simulink model "sampleModel1507_5_sub"  (R2023a)
settings: Solver=VariableStepAuto  StartTime=0.0  StopTime=10.0  RelTol=1e-3
libraries: hdlsllib x8, simulink x3
settings Model: Creator=user1  LastModifiedBy=user1
settings OptimizationCC: BlockReduction=off  ConditionallyExecuteInputs=off

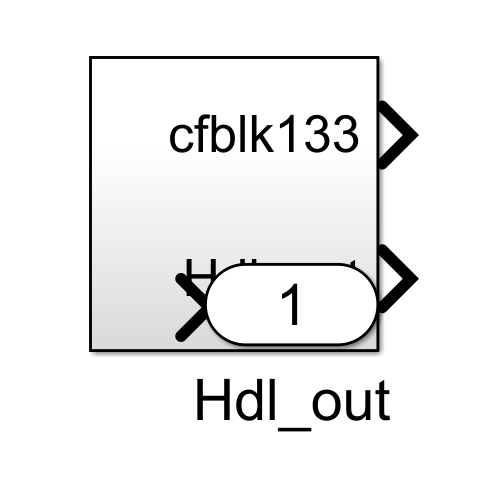
[thumbnail: Simulink's stored preview of the top-level diagram]
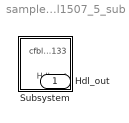
== system sampleModel1507_5_sub ==
  Subsystem : Subsystem
  Hdl_out : Outport  OutDataTypeStr=uint8

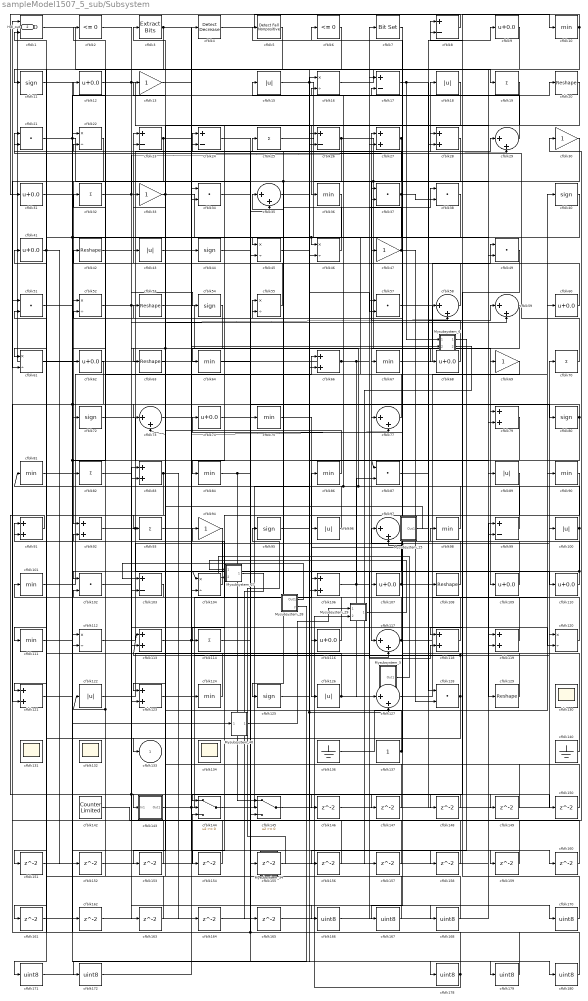
== system sampleModel1507_5_sub/Subsystem ==
  Mysubsystem_15 : Subsystem  TreatAsAtomicUnit=on  RTWFcnName=Mysubsystem_15
      settings: RTWFcnNameOpts=User specified  RTWFileNameOpts=Use function name
  Mysubsystem_27 : Subsystem  TreatAsAtomicUnit=on  RTWFcnName=Mysubsystem_27
      settings: RTWFcnNameOpts=User specified  RTWFileNameOpts=Use function name
  Mysubsystem_28 : Subsystem  TreatAsAtomicUnit=on  RTWFcnName=Mysubsystem_28
      settings: RTWFcnNameOpts=User specified  RTWFileNameOpts=Use function name
  Mysubsystem_29 : Subsystem  TreatAsAtomicUnit=on  RTWFcnName=Mysubsystem_29
      settings: RTWFcnNameOpts=User specified  RTWFileNameOpts=Use function name
  Mysubsystem_34 : Subsystem  TreatAsAtomicUnit=on  RTWFcnName=Mysubsystem_34
      settings: RTWFcnNameOpts=User specified  RTWFileNameOpts=Use function name
  Mysubsystem_40 : Subsystem  TreatAsAtomicUnit=on  RTWFcnName=Mysubsystem_40
      settings: RTWFcnNameOpts=User specified  RTWFileNameOpts=Use function name
  Mysubsystem_5 : Subsystem  TreatAsAtomicUnit=on  RTWFcnName=Mysubsystem_5
      settings: RTWFcnNameOpts=User specified  RTWFileNameOpts=Use function name
  Mysubsystem_6 : Subsystem  TreatAsAtomicUnit=on  RTWFcnName=Mysubsystem_6
      settings: RTWFcnNameOpts=User specified  RTWFileNameOpts=Use function name
  cfblk1 : Logic  AllPortsSameDT=off  OutDataTypeStr=boolean
  cfblk{10,36,64,67,75,81,84,86,90,98,101,111,124} (13 alike) : MinMax  OutDataTypeStr=uint8
  cfblk{15,18,43,89,96,100,122,126} (8 alike) : Abs  OutDataTypeStr=uint8  SaturateOnIntegerOverflow=off
  cfblk{21,34,37..38,49,51,57,87,102,128} (10 alike) : DotProduct  OutDataTypeStr=uint8
  cfblk{8,17,23..24,26,99,103} (7 alike) : Sum  Inputs=+-  OutDataTypeStr=uint8
  cfblk{16,22,45..46,52,55,61,104,112,120} (10 alike) : Product  Inputs=*/  OutDataTypeStr=uint8  RndMeth=Zero  SaturateOnIntegerOverflow=on
  cfblk{27..28,66,79,83,91..92,106,113,118..119,121,123} (13 alike) : Sum  OutDataTypeStr=uint8
  cfblk{9,12,31,41,60,62,68,74,107,109..110,116} (12 alike) : Bias  Bias=0.0  SaturateOnIntegerOverflow=off
  cfblk{20,42,53,63,108,129} (6 alike) : Reshape
  cfblk{11,40,44,54,72,80,95,125} (8 alike) : Signum
  cfblk{19,25,32,70,82,93,114} (7 alike) : Sum  Inputs=+  OutDataTypeStr=uint8
  cfblk{29,35,58..59,73,77,97,117,127} (9 alike) : Sum  Inputs=|++  OutDataTypeStr=uint8
  cfblk{13,30,33,47,69,94} (6 alike) : Gain  OutDataTypeStr=uint8
  cfblk{130..132,134} (4 alike) : Scope
      settings: Floating=on
  cfblk136 : Ground
  cfblk137 : Constant  OutDataTypeStr=uint8  SampleTime=-1
  cfblk140 : Ground
  cfblk142 : hdlsllib/Sources/Counter Limited  uplimit=7  tsamp=-1
  cfblk143 : Subsystem
      settings: LibrarySourceBlock=|
      | hdlsllib/Ports &
      | Subsystems/Subsystem
  cfblk144 : Switch  OutDataTypeStr=uint8  SaturateOnIntegerOverflow=off  InputSameDT=off
  cfblk145 : Switch  OutDataTypeStr=uint8  SaturateOnIntegerOverflow=off  InputSameDT=off
  cfblk{146..165} (20 alike) : Delay  SampleTime=1
  cfblk{166..168,170..172,178..180} (9 alike) : DataTypeConversion  OutDataTypeStr=uint8  SaturateOnIntegerOverflow=off  RndMeth=Floor
  cfblk2 : hdlsllib/Logic and Bit Operations/Compare To Zero  relop=<=  OutDataTypeStr=uint8
  cfblk3 : simulink/Logic and Bit Operations/Extract Bits  bitsToExtract=Upper half  numBits=8  bitIdxRange=[0 7]  outScalingMode=Preserve fixed-point scaling
      settings: LibrarySourceBlock=|
      | hdlsllib/Logic and Bit
      | Operations/Extract Bits
  cfblk4 : simulink/Logic and Bit Operations/Detect Decrease  vinit=0.0  OutDataTypeStr=uint8
      settings: LibrarySourceBlock=|
      | hdlsllib/Logic and Bit
      | Operations/Detect
      | Decrease
  cfblk5 : hdlsllib/Logic and Bit Operations/Detect Fall Nonpositive  vinit=0  OutDataTypeStr=uint8
  cfblk6 : hdlsllib/Logic and Bit Operations/Compare To Zero  relop=<=  OutDataTypeStr=uint8
  cfblk7 : simulink/Logic and Bit Operations/Bit Set  iBit=0
      settings: LibrarySourceBlock=|
      | hdlsllib/Logic and Bit
      | Operations/Bit Set
  cfblk133 : Outport  OutDataTypeStr=uint8  VectorParamsAs1DForOutWhenUnconnected=off
  Hdl_out : Outport  Port=2  OutDataTypeStr=uint8
  wires:
  cfblk67/1 -> cfblk49/1
  cfblk101/1 -> cfblk66/1
  cfblk66/1 -> Hdl_out/1, cfblk38/1, cfblk127/1
  cfblk113/1 -> cfblk158/1, Mysubsystem_6/2(In2)
  cfblk55/1 -> cfblk23/1
  cfblk29/1 -> cfblk15/1
  cfblk99/1 -> cfblk55/2, cfblk64/1
  cfblk83/1 -> cfblk171/1, cfblk164/1
  cfblk26/1 -> cfblk103/2, cfblk79/2, cfblk68/1
  cfblk98/1 -> cfblk16/2, cfblk81/1
  cfblk102/1 -> cfblk166/1, cfblk145/3
  cfblk69/1 -> cfblk45/1
  cfblk47/1 -> cfblk128/2, cfblk21/1
  cfblk38/1 -> cfblk121/1, cfblk46/1
  cfblk57/1 -> cfblk109/1
  cfblk52/1 -> cfblk58/2, cfblk24/1
  cfblk110/1 -> cfblk37/2, cfblk104/1
  cfblk16/1 -> cfblk19/1
  cfblk22/1 -> cfblk92/1
  cfblk92/1 -> cfblk117/2, cfblk18/1
  cfblk100/1 -> cfblk154/1, cfblk37/1
  cfblk145/1 -> cfblk70/1
  cfblk112/1 -> cfblk100/1
  cfblk128/1 -> cfblk161/1, cfblk5/1, cfblk113/1
  cfblk3/1 -> cfblk82/1, cfblk44/1
  cfblk61/1 -> cfblk87/1, Mysubsystem_40/1(In1)
  cfblk80/1 -> cfblk106/2, cfblk72/1
  cfblk129/1 -> cfblk97/2, cfblk42/1
  cfblk75/1 -> cfblk126/1
  cfblk96/1 -> cfblk12/1
  cfblk8/1 -> cfblk31/1
  cfblk70/1 -> cfblk21/2
  cfblk40/1 -> cfblk46/2
  cfblk9/1 -> cfblk66/2
  cfblk116/1 -> cfblk35/1
  cfblk104/1 -> cfblk91/1
  cfblk33/1 -> cfblk73/1, cfblk45/2
  cfblk124/1 -> cfblk32/1
  cfblk127/1 -> cfblk60/1
  cfblk109/1 -> cfblk6/1
  cfblk5/1 -> cfblk11/1
  cfblk123/1 -> cfblk120/1
  cfblk21/1 -> cfblk20/1, cfblk75/1
  cfblk12/1 -> cfblk54/1, cfblk89/1
  cfblk107/1 -> cfblk96/1, cfblk58/1
  cfblk25/1 -> cfblk129/1
  cfblk143/1(Out1) -> cfblk77/2, cfblk86/1
  cfblk20/1 -> cfblk36/1
  cfblk62/1 -> cfblk121/2, cfblk112/2
  cfblk28/1 -> cfblk83/2
  cfblk95/1 -> cfblk168/1
  cfblk97/1 -> cfblk9/1, cfblk102/1
  cfblk126/1 -> cfblk118/2, cfblk41/1
  cfblk15/1 -> cfblk57/2, cfblk117/1
  cfblk18/1 -> cfblk84/1
  cfblk87/1 -> cfblk59/1
  cfblk1/1 -> cfblk99/2
  cfblk89/1 -> cfblk114/1
  cfblk41/1 -> cfblk152/1, cfblk151/1
  cfblk10/1 -> cfblk111/1, cfblk8/1
  cfblk31/1 -> cfblk149/1, cfblk49/2
  cfblk35/1 -> cfblk110/1
  cfblk68/1 -> cfblk27/1
  cfblk91/1 -> cfblk143/1(In1)
  cfblk43/1 -> cfblk4/1
  cfblk27/1 -> cfblk77/1, cfblk125/1, cfblk133/1
  cfblk74/1 -> cfblk116/1
  cfblk63/1 -> cfblk13/1
  cfblk118/1 -> cfblk94/1
  cfblk6/1 -> cfblk61/1
  cfblk17/1 -> cfblk108/1, Mysubsystem_6/1(In1)
  cfblk82/1 -> cfblk113/2
  cfblk19/1 -> cfblk63/1
  cfblk122/1 -> cfblk57/1
  cfblk144/1 -> cfblk26/2
  cfblk108/1 -> cfblk74/1
  cfblk86/1 -> cfblk52/2
  cfblk120/1 -> cfblk106/1
  cfblk58/1 -> cfblk25/1
  cfblk103/1 -> cfblk102/2
  cfblk72/1 -> cfblk119/2
  cfblk119/1 -> cfblk55/1
  cfblk51/1 -> cfblk178/1
  cfblk13/1 -> cfblk69/1
  cfblk142/1 -> cfblk30/1
  cfblk36/1 -> cfblk62/1
  cfblk84/1 -> cfblk145/1, cfblk28/1
  cfblk73/1 -> cfblk124/1
  cfblk125/1 -> cfblk180/1, cfblk127/2
  cfblk42/1 -> cfblk59/2
  cfblk23/1 -> cfblk61/2, cfblk144/2
  cfblk64/1 -> cfblk80/1
  cfblk53/1 -> cfblk128/1
  cfblk46/1 -> cfblk24/2
  cfblk4/1 -> cfblk10/1
  cfblk30/1 -> cfblk107/1
  cfblk45/1 -> cfblk17/2
  cfblk59/1 -> cfblk67/1
  cfblk140/1 -> cfblk53/1
  cfblk60/1 -> cfblk47/1
  cfblk117/1 -> cfblk101/1, cfblk40/1
  cfblk77/1 -> cfblk2/1
  cfblk137/1 -> cfblk97/1, cfblk33/1
  cfblk37/1 -> cfblk93/1, cfblk38/2, cfblk3/1
  cfblk24/1 -> cfblk79/1
  cfblk106/1 -> cfblk87/2, cfblk29/1
  cfblk32/1 -> cfblk120/2, cfblk29/2
  cfblk90/1 -> cfblk118/1
  cfblk54/1 -> cfblk73/2, cfblk123/2
  cfblk136/1 -> cfblk90/1
  cfblk81/1 -> cfblk146/1
  cfblk146/1 -> cfblk28/2
  cfblk79/1 -> cfblk147/1
  cfblk147/1 -> cfblk26/1
  cfblk49/1 -> cfblk148/1
  cfblk148/1 -> cfblk144/1
  cfblk149/1 -> cfblk8/2
  cfblk111/1 -> cfblk150/1
  cfblk150/1 -> cfblk23/2
  cfblk151/1 -> cfblk104/2
  cfblk152/1 -> cfblk144/3
  cfblk94/1 -> cfblk153/1
  cfblk153/1 -> cfblk92/2
  cfblk154/1 -> cfblk52/1
  cfblk44/1 -> cfblk155/1
  cfblk155/1 -> cfblk99/1
  cfblk156/1 -> cfblk1/1
  cfblk157/1 -> cfblk112/1
  cfblk158/1 -> cfblk16/1
  cfblk121/1 -> cfblk159/1
  cfblk159/1 -> cfblk91/2
  cfblk93/1 -> cfblk160/1
  cfblk160/1 -> cfblk83/1
  cfblk161/1 -> cfblk35/2
  cfblk11/1 -> cfblk162/1
  cfblk162/1 -> cfblk17/1
  cfblk2/1 -> cfblk163/1
  cfblk163/1 -> cfblk1/2
  cfblk164/1 -> cfblk27/2
  cfblk165/1 -> cfblk119/1
  cfblk166/1 -> cfblk7/1
  cfblk7/1 -> cfblk167/1
  cfblk167/1 -> cfblk43/1
  cfblk168/1 -> cfblk122/1, cfblk22/2
  cfblk34/1 -> cfblk170/1
  cfblk170/1 -> cfblk98/1
  cfblk171/1 -> cfblk34/1
  cfblk172/1 -> cfblk34/2
  cfblk178/1 -> cfblk22/1, cfblk145/2, Mysubsystem_29/2(In2)
  cfblk114/1 -> cfblk179/1
  cfblk179/1 -> cfblk51/1
  cfblk180/1 -> cfblk51/2
  Mysubsystem_6/1(Out1) -> cfblk156/1
  Mysubsystem_6/2(Out2) -> cfblk157/1
  Mysubsystem_15/1(Out1) -> cfblk123/1
  Mysubsystem_5/1(Out1) -> Mysubsystem_27/2(In2)
  Mysubsystem_27/1(Out1) -> cfblk165/1
  Mysubsystem_28/1(Out1) -> cfblk103/1
  Mysubsystem_28/2(y) -> cfblk172/1
  Mysubsystem_29/1(Out1) -> Mysubsystem_27/1(In1)
  Mysubsystem_34/1(Out1) -> cfblk95/1
  Mysubsystem_40/1(Out1) -> Mysubsystem_29/1(In1)

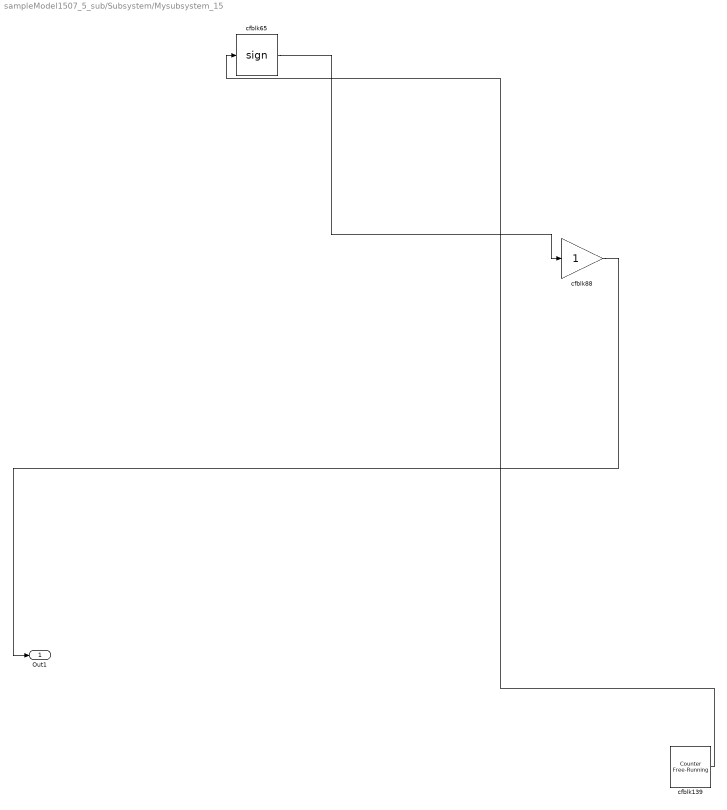
== system sampleModel1507_5_sub/Subsystem/Mysubsystem_15 ==
  cfblk139 : hdlsllib/Sources/Counter Free-Running  NumBits=16  tsamp=-1
  cfblk65 : Signum
  cfblk88 : Gain
  Out1 : Outport
  wires:
  cfblk65/1 -> cfblk88/1
  cfblk139/1 -> cfblk65/1
  cfblk88/1 -> Out1/1

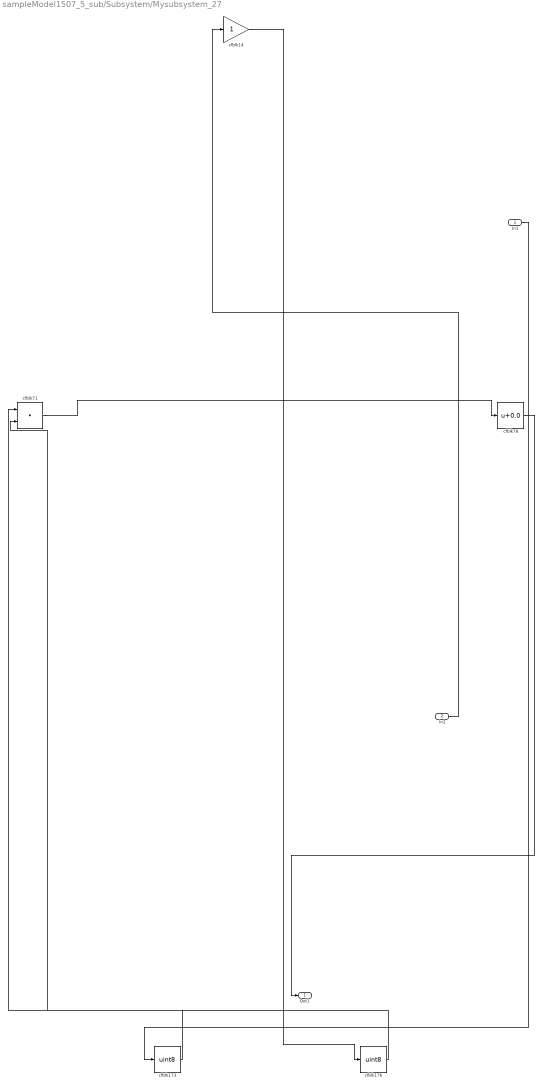
== system sampleModel1507_5_sub/Subsystem/Mysubsystem_27 ==
  In1 : Inport
  In2 : Inport  Port=2
  cfblk14 : Gain
  cfblk173 : DataTypeConversion  OutDataTypeStr=uint8  SaturateOnIntegerOverflow=off  RndMeth=Floor
  cfblk176 : DataTypeConversion  OutDataTypeStr=uint8  SaturateOnIntegerOverflow=off  RndMeth=Floor
  cfblk71 : DotProduct  OutDataTypeStr=Inherit: Inherit via internal rule
  cfblk78 : Bias  Bias=0.0  SaturateOnIntegerOverflow=off
  Out1 : Outport
  wires:
  In1/1 -> cfblk173/1
  cfblk176/1 -> cfblk71/2
  cfblk173/1 -> cfblk71/1
  In2/1 -> cfblk14/1
  cfblk14/1 -> cfblk176/1
  cfblk78/1 -> Out1/1
  cfblk71/1 -> cfblk78/1

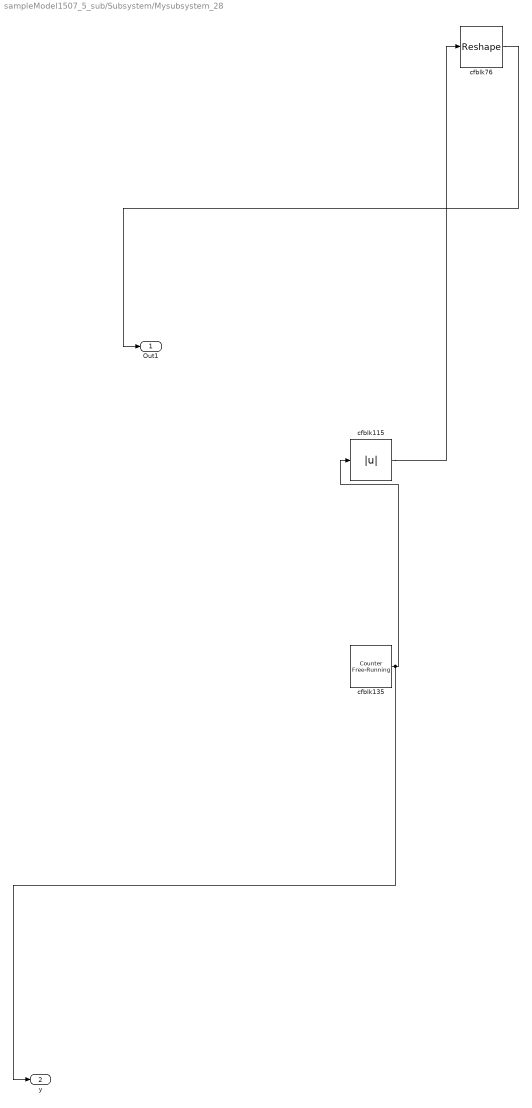
== system sampleModel1507_5_sub/Subsystem/Mysubsystem_28 ==
  cfblk115 : Abs  SaturateOnIntegerOverflow=off
  cfblk135 : hdlsllib/Sources/Counter Free-Running  NumBits=16  tsamp=-1
  cfblk76 : Reshape
  Out1 : Outport
  y : Outport  Port=2
  wires:
  cfblk76/1 -> Out1/1
  cfblk135/1 -> cfblk115/1, y/1
  cfblk115/1 -> cfblk76/1

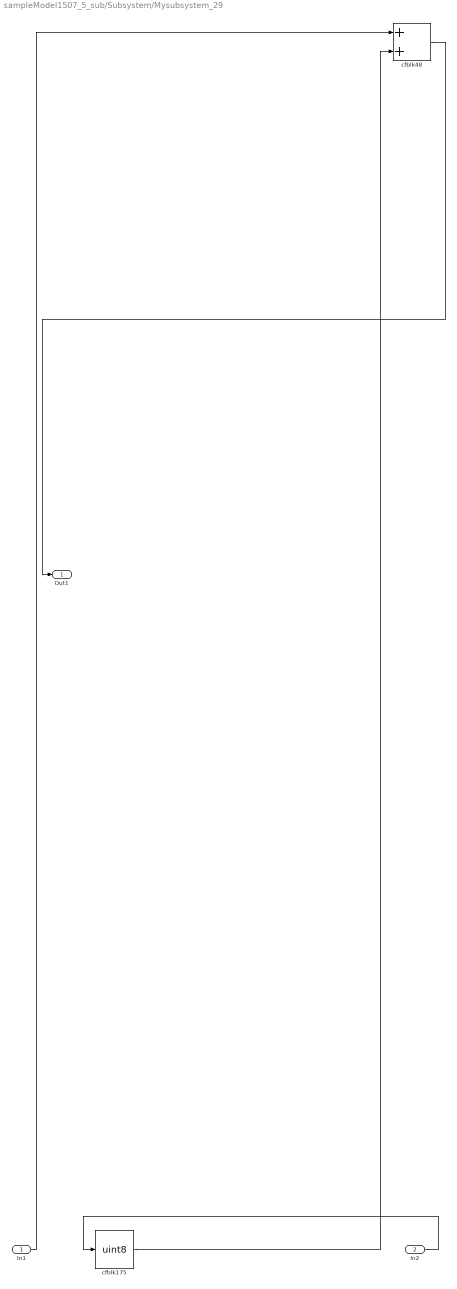
== system sampleModel1507_5_sub/Subsystem/Mysubsystem_29 ==
  In1 : Inport
  In2 : Inport  Port=2
  cfblk175 : DataTypeConversion  OutDataTypeStr=uint8  SaturateOnIntegerOverflow=off  RndMeth=Floor
  cfblk48 : Sum
  Out1 : Outport
  wires:
  In2/1 -> cfblk175/1
  In1/1 -> cfblk48/1
  cfblk175/1 -> cfblk48/2
  cfblk48/1 -> Out1/1

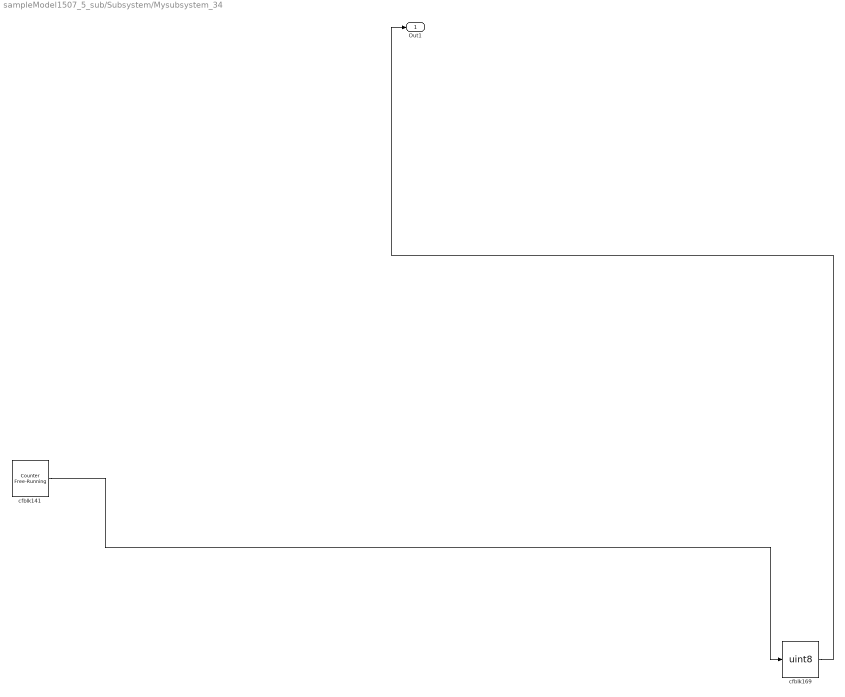
== system sampleModel1507_5_sub/Subsystem/Mysubsystem_34 ==
  cfblk141 : hdlsllib/Sources/Counter Free-Running  NumBits=16  tsamp=-1
  cfblk169 : DataTypeConversion  OutDataTypeStr=uint8  SaturateOnIntegerOverflow=off  RndMeth=Floor
  Out1 : Outport
  wires:
  cfblk169/1 -> Out1/1
  cfblk141/1 -> cfblk169/1

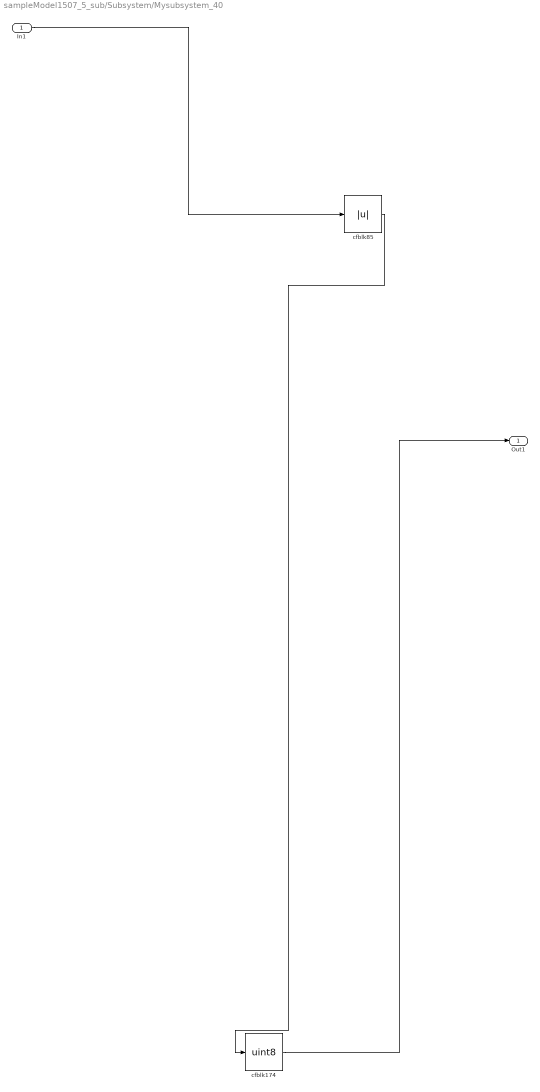
== system sampleModel1507_5_sub/Subsystem/Mysubsystem_40 ==
  In1 : Inport
  cfblk174 : DataTypeConversion  OutDataTypeStr=uint8  SaturateOnIntegerOverflow=off  RndMeth=Floor
  cfblk85 : Abs  SaturateOnIntegerOverflow=off
  Out1 : Outport
  wires:
  cfblk174/1 -> Out1/1
  cfblk85/1 -> cfblk174/1
  In1/1 -> cfblk85/1

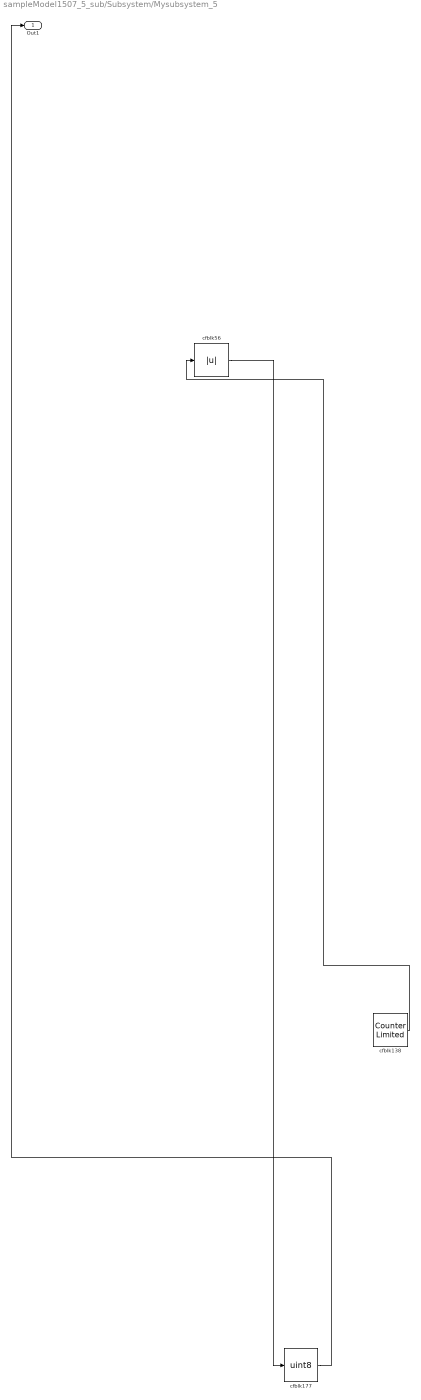
== system sampleModel1507_5_sub/Subsystem/Mysubsystem_5 ==
  cfblk138 : hdlsllib/Sources/Counter Limited  uplimit=7  tsamp=-1
  cfblk177 : DataTypeConversion  OutDataTypeStr=uint8  SaturateOnIntegerOverflow=off  RndMeth=Floor
  cfblk56 : Abs  SaturateOnIntegerOverflow=off
  Out1 : Outport
  wires:
  cfblk177/1 -> Out1/1
  cfblk56/1 -> cfblk177/1
  cfblk138/1 -> cfblk56/1

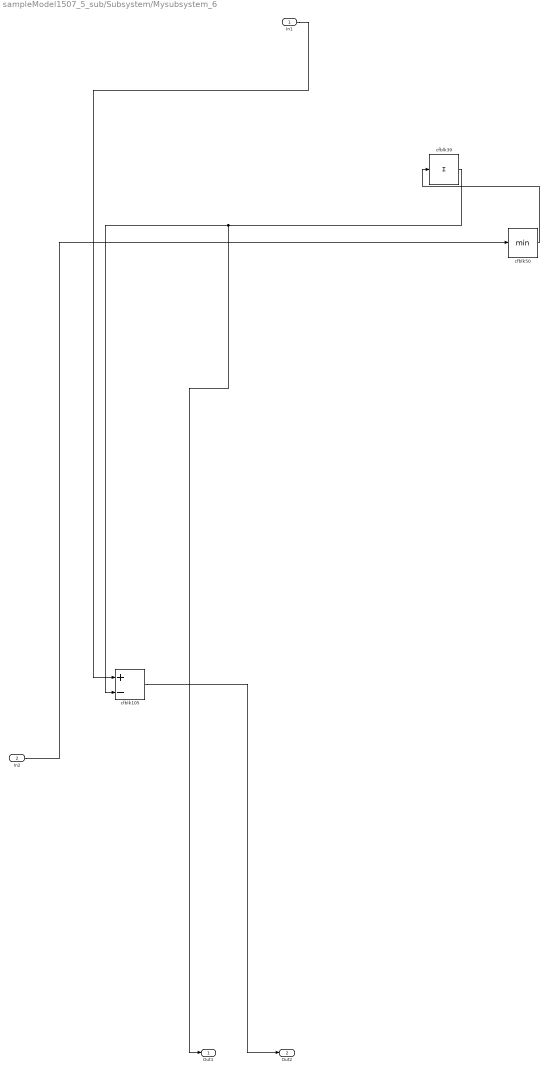
== system sampleModel1507_5_sub/Subsystem/Mysubsystem_6 ==
  In1 : Inport
  In2 : Inport  Port=2
  cfblk105 : Sum  Inputs=+-
  cfblk39 : Sum  Inputs=+
  cfblk50 : MinMax
  Out1 : Outport
  Out2 : Outport  Port=2
  wires:
  In2/1 -> cfblk50/1
  cfblk39/1 -> cfblk105/2, Out1/1
  cfblk105/1 -> Out2/1
  In1/1 -> cfblk105/1
  cfblk50/1 -> cfblk39/1

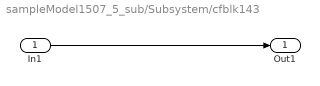
== system sampleModel1507_5_sub/Subsystem/cfblk143 ==
  In1 : Inport
  Out1 : Outport
  wires:
  In1/1 -> Out1/1
